simulink model "nonlinmodel"  (R2025a)
settings: Solver=VariableStepAuto  StartTime=0.0  StopTime=1  RelTol=1e-3
values from neighbouring files (symbols this model uses):
  k = lqr(A, B, Q, R)    [determineABK.m]
  r = [0;0;0;0]    [determineABK.m]
  xs = [0;0;0;0]    [determineABK.m]    (also in simulate_sys.m)
settings Model: Creator=quintenpienaar  LastModifiedBy=quintenpienaar
settings DataIOCC: SaveOutput=off  SignalLogging=off  DSMLogging=off  SaveTime=off  ReturnWorkspaceOutputs=off

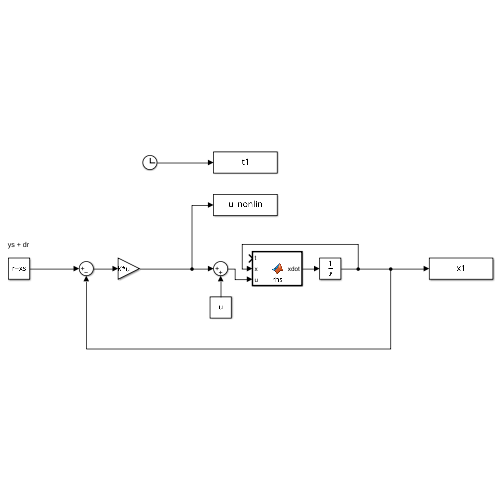
[thumbnail: Simulink's stored preview of the top-level diagram]
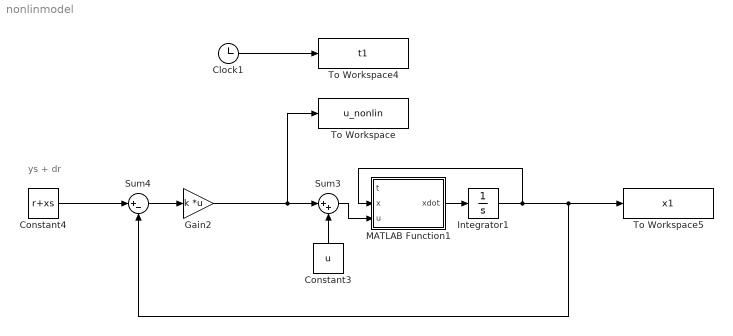
== system nonlinmodel ==
  note: ys + dr
  Clock1 : Clock
  Constant3 : Constant  Value=u
  Constant4 : Constant  Value=r+xs
  Gain2 : Gain  Gain=k  Multiplication=Matrix(K*u)
  Integrator1 : Integrator  InitialCondition=[0;0;deg2rad(10);0]
  MATLAB Function1 : MATLAB Function  TreatAsAtomicUnit=on
  Sum3 : Sum  Inputs=|++
  Sum4 : Sum  Inputs=|+-
  To Workspace : ToWorkspace  VariableName=u_nonlin  SampleTime=-1
      settings: Save2DSignal=2-D array (concatenate along first dimension)
  To Workspace4 : ToWorkspace  VariableName=t1  SampleTime=-1
      settings: Save2DSignal=2-D array (concatenate along first dimension)
  To Workspace5 : ToWorkspace  VariableName=x1  SampleTime=-1
      settings: Save2DSignal=2-D array (concatenate along first dimension)
  wires:
  Sum3/1 -> MATLAB Function1/3(u)
  Constant4/1 -> Sum4/1
  Constant3/1 -> Sum3/2
  Sum4/1 -> Gain2/1
  MATLAB Function1/1(xdot) -> Integrator1/1
  Clock1/1 -> To Workspace4/1
  Integrator1/1 -> MATLAB Function1/2(x), Sum4/2, To Workspace5/1
  Gain2/1 -> To Workspace/1, Sum3/1

== matlab function nonlinmodel/MATLAB Function1 ==
  data: t input; x input; u input; xdot output
function xdot = rhs(t, x, u)

g = 9.81;
l = 0.019;      % segway: without battery
mp = 0.068;      % kg without batteries (does not include wheels)
mw = 0.034;      % verified 2 wheels and axle
rw = 0.022;      % 44/2 = radius of wheel in m (small wheel)
Iw = 1/2 * mw * rw^2;   % uniform disk
rm = 13;
kb = 0.155;
kt = 0.1;

Tm = (kt/rm)*(u+((kb/rw)*x(2))+(kb*x(4)));

xdot = zeros(4, 1);

xdot(1) = x(2);
xdot(3) = x(4);

alpha = x(3);
alphad = x(4);

% looking for alphadd xdot(4) and xdd xdot(2)

A = [0 0 0 0 0 1 1;
    -mw 0 0 -1 1 0 0;
    0 0 Iw rw 0 0 0;
    -mp mp*l*cos(alpha) 0 0 -1 0 0;
    0 mp*l*sin(alpha) 0 0 0 -1 0;
    0 0 0 0 -l*cos(alpha) -l*sin(alpha) 0;
    1 0 rw 0 0 0 0];

b = [mw*g;
    0;
    Tm;
    mp*l*(alphad^2)*sin(alpha);
    ((mp*g)-(l*(alphad^2)*cos(alpha)));
    Tm
    Tm];

z = A\b;

xdot(2) = z(1);
xdot(4) = z(2);
end
